simulink library "dlbsBlockLog"  (R2025b)
settings: Solver=VariableStepAuto  StartTime=0.0  StopTime=10.0  RelTol=1e-3
libraries: dlbsBlockExtractGradientGF x1, dlbsBlockInsertGradientGF x1
settings Model: Creator=lt6037  LastModifiedBy=lt6037

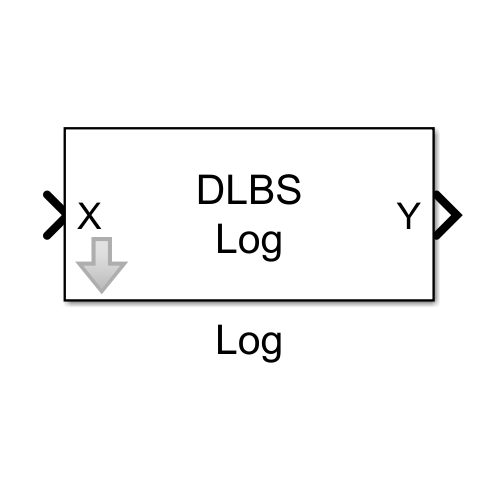
[thumbnail: Simulink's stored preview of the top-level diagram]
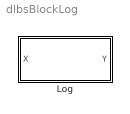
== system dlbsBlockLog ==
  Log : Subsystem
      mask help: Applies the natural logarithm to the input tensor. The operation is applied element-wise across all tensor elements.
      mask Help: web("dlbsHelpBlockLog.html")
      mask Display: fprintf("DLBS\nLog")

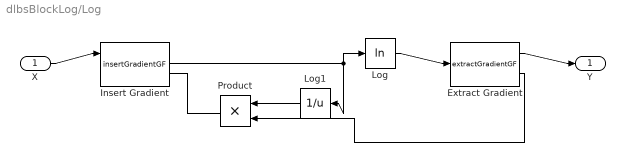
== system dlbsBlockLog/Log ==
  X : Inport
  Extract Gradient : dlbsBlockExtractGradientGF/extractGradientGF
  Insert Gradient : dlbsBlockInsertGradientGF/insertGradientGF
  Log : Math  Operator=log
  Log1 : Math  Operator=reciprocal
  Product : Product
  Y : Outport
  wires:
  Insert Gradient/1 -> Log1/1, Log/1
  Log1/1 -> Product/1
  Extract Gradient/2 -> Product/2
  Log/1 -> Extract Gradient/1
  Product/1 -> Insert Gradient/2
  X/1 -> Insert Gradient/1
  Extract Gradient/1 -> Y/1
